simulink model "main"  (R2022a)
settings: Solver=FixedStepDiscrete  StartTime=0.0  StopTime=Inf  FixedStep=(50e-6)-(sim_en*4.995e-5)  RelTol=1e-3  EnableMultiTasking=on
model workspace (MAT data in the model file):
  Param : Simulink.Parameter (value not decoded)
  ac_ok : Simulink.Signal (value not decoded)
  ac_ok_120 : Simulink.Signal (value not decoded)
  bulk_voltage : Simulink.Signal (value not decoded)
  burstduty_integ_max : Simulink.Signal (value not decoded)
  burstduty_integ_min : Simulink.Signal (value not decoded)
  burstduty_ki : Simulink.Signal (value not decoded)
  burstduty_kp : Simulink.Signal (value not decoded)
  calib_ok : Simulink.Signal (value not decoded)
  can_addr1 : Simulink.Signal (value not decoded)
  can_addr2 : Simulink.Signal (value not decoded)
  can_addr3 : Simulink.Signal (value not decoded)
  can_addr4 : Simulink.Signal (value not decoded)
  can_data_rx : Simulink.Signal (value not decoded)
  can_data_tx : Simulink.Signal (value not decoded)
  can_timeout_120 : Simulink.Signal (value not decoded)
  chksum_scircv : Simulink.Signal (value not decoded)
  clllc_en_120 : Simulink.Signal (value not decoded)
  clllc_fault_120 : Simulink.Signal (value not decoded)
  clllc_ok_120 : Simulink.Signal (value not decoded)
  cmpss1h : Simulink.Signal (value not decoded)
  cmpss1l : Simulink.Signal (value not decoded)
  cmpss2h : Simulink.Signal (value not decoded)
  cmpss2l : Simulink.Signal (value not decoded)
  cmpss3h : Simulink.Signal (value not decoded)
  cmpss3l : Simulink.Signal (value not decoded)
  cmpss4h : Simulink.Signal (value not decoded)
  cmpss4l : Simulink.Signal (value not decoded)
  cmpss5h : Simulink.Signal (value not decoded)
  cmpss5l : Simulink.Signal (value not decoded)
  cmpss6h : Simulink.Signal (value not decoded)
  cmpss6l : Simulink.Signal (value not decoded)
  cmpss7h : Simulink.Signal (value not decoded)
  cmpss7l : Simulink.Signal (value not decoded)
  cmpss8h : Simulink.Signal (value not decoded)
  cmpss8l : Simulink.Signal (value not decoded)
  cnt_idle : Simulink.Signal (value not decoded)
  cnt_orps : Simulink.Signal (value not decoded)
  cnt_scircv : Simulink.Signal (value not decoded)
  cnt_scixmt : Simulink.Signal (value not decoded)
  cnt_scixmt_func : Simulink.Signal (value not decoded)
  cnt_temp_mux : Simulink.Signal (value not decoded)
  cnt_vdroop : Simulink.Signal (value not decoded)
  config_ok : Simulink.Signal (value not decoded)
  control_en : Simulink.Signal (value not decoded)
  cp_ready_120 : Simulink.Signal (value not decoded)
  d2d_en : Simulink.Signal (value not decoded)
  dchg_off : Simulink.Signal (value not decoded)
  debug_dacb : Simulink.Signal (value not decoded)
  debug_dacc : Simulink.Signal (value not decoded)
  debug_msg1 : Simulink.Signal (value not decoded)
  debug_msg2 : Simulink.Signal (value not decoded)
  debug_msg3 : Simulink.Signal (value not decoded)
  debug_msg4 : Simulink.Signal (value not decoded)
  debug_msg5 : Simulink.Signal (value not decoded)
  debug_msg6 : Simulink.Signal (value not decoded)
  dir_v2g : Simulink.Signal (value not decoded)
  eoss_llc1 : Simulink.Signal (value not decoded)
  eoss_llc2 : Simulink.Signal (value not decoded)
  eoss_orps : Simulink.Signal (value not decoded)
  fault_ocp : Simulink.Signal (value not decoded)
  fault_otp : Simulink.Signal (value not decoded)
  fault_ovp : Simulink.Signal (value not decoded)
  fut_en : Simulink.Signal (value not decoded)
  fwd_en_120 : Simulink.Signal (value not decoded)
  gain_llc1_sec_idc : Simulink.Signal (value not decoded)
  gain_llc1_temp_sr : Simulink.Signal (value not decoded)
  gain_llc2_sec_idc : Simulink.Signal (value not decoded)
  gain_vbat : Simulink.Signal (value not decoded)
  gain_vbulk : Simulink.Signal (value not decoded)
  gain_vout : Simulink.Signal (value not decoded)
  input_current_phasea : Simulink.Signal (value not decoded)
  input_current_phaseb : Simulink.Signal (value not decoded)
  input_current_phasec : Simulink.Signal (value not decoded)
  input_freq : Simulink.Signal (value not decoded)
  input_power : Simulink.Signal (value not decoded)
  input_voltage_phasea : Simulink.Signal (value not decoded)
  input_voltage_phaseb : Simulink.Signal (value not decoded)
  input_voltage_phasec : Simulink.Signal (value not decoded)
  ishare_arbiter : Simulink.Signal (value not decoded)
  ishare_thresh : Simulink.Signal (value not decoded)
  led_g : Simulink.Signal (value not decoded)
  led_r : Simulink.Signal (value not decoded)
  led_y : Simulink.Signal (value not decoded)
  llc1_burst_integ : Simulink.Signal (value not decoded)
  llc1_burstduty_buffer : Simulink.Signal (value not decoded)
  llc1_pfm_error : Simulink.Signal (value not decoded)
  llc1_pfm_integ : Simulink.Signal (value not decoded)
  llc1_pfm_prop : Simulink.Signal (value not decoded)
  llc1_pri_idc : Simulink.Signal (value not decoded)
  llc1_ps_buffer : Simulink.Signal (value not decoded)
  llc1_pspwm_error : Simulink.Signal (value not decoded)
  llc1_pspwm_integ : Simulink.Signal (value not decoded)
  llc1_pspwm_prop : Simulink.Signal (value not decoded)
  llc1_sec_idc : Simulink.Signal (value not decoded)
  llc1_temp_sr : Simulink.Signal (value not decoded)
  llc1_ts_tbctr_buffer : Simulink.Signal (value not decoded)
  llc2_burst_integ : Simulink.Signal (value not decoded)
  llc2_burstduty_buffer : Simulink.Signal (value not decoded)
  llc2_en : Simulink.Signal (value not decoded)
  llc2_en_buffer : Simulink.Signal (value not decoded)
  llc2_pfm_error : Simulink.Signal (value not decoded)
  llc2_pfm_integ : Simulink.Signal (value not decoded)
  llc2_pfm_prop : Simulink.Signal (value not decoded)
  llc2_pri_idc : Simulink.Signal (value not decoded)
  llc2_ps_buffer : Simulink.Signal (value not decoded)
  llc2_pspwm_error : Simulink.Signal (value not decoded)
  llc2_pspwm_integ : Simulink.Signal (value not decoded)
  llc2_pspwm_prop : Simulink.Signal (value not decoded)
  llc2_sec_idc : Simulink.Signal (value not decoded)
  llc2_temp_sr : Simulink.Signal (value not decoded)
  llc2_ts_tbctr_buffer : Simulink.Signal (value not decoded)
  loop_adcint : Simulink.Signal (value not decoded)
  loop_control : Simulink.Signal (value not decoded)
  loop_idle : Simulink.Signal (value not decoded)
  mid_bulk_voltage : Simulink.Signal (value not decoded)
  mode_120 : Simulink.Signal (value not decoded)
  mode_cc_cv : Simulink.Signal (value not decoded)
  myParam : mpt.Parameter (value not decoded)
  obc_ok_120 : Simulink.Signal (value not decoded)
  offset_llc1_sec_idc : Simulink.Signal (value not decoded)
  offset_llc1_temp_sr : Simulink.Signal (value not decoded)
  offset_llc2_sec_idc : Simulink.Signal (value not decoded)
  offset_vbat : Simulink.Signal (value not decoded)
  offset_vbulk : Simulink.Signal (value not decoded)
  offset_vout : Simulink.Signal (value not decoded)
  openloop_en : Simulink.Signal (value not decoded)
  openloop_fault_en : Simulink.Signal (value not decoded)
  ot_fault_120 : Simulink.Signal (value not decoded)
  pfc_en : Simulink.Signal (value not decoded)
  pfc_en_120 : Simulink.Signal (value not decoded)
  pfc_fw_revision : Simulink.Signal (value not decoded)
  pfc_fw_revision_bootloader : Simulink.Signal (value not decoded)
  pfc_fw_revision_debug : Simulink.Signal (value not decoded)
  pfc_ok : Simulink.Signal (value not decoded)
  pfc_ok_120 : Simulink.Signal (value not decoded)
  pfm_a0 : Simulink.Signal (value not decoded)
  pfm_a1 : Simulink.Signal (value not decoded)
  pfm_integ_max : Simulink.Signal (value not decoded)
  pfm_integ_min : Simulink.Signal (value not decoded)
  pfm_ki : Simulink.Signal (value not decoded)
  pfm_kp : Simulink.Signal (value not decoded)
  pri_fut_en : Simulink.Signal (value not decoded)
  pri_fut_en_buffer : Simulink.Signal (value not decoded)
  pri_halfbridge_en : Simulink.Signal (value not decoded)
  pri_halfbridge_en_buffer : Simulink.Signal (value not decoded)
  pspwm_integ_max : Simulink.Signal (value not decoded)
  pspwm_integ_min : Simulink.Signal (value not decoded)
  pspwm_ki : Simulink.Signal (value not decoded)
  pspwm_kp : Simulink.Signal (value not decoded)
  ref_idclink_max : Simulink.Signal (value not decoded)
  ref_iout : Simulink.Signal (value not decoded)
  ref_iout_calib : Simulink.Signal (value not decoded)
  ref_iout_llc1 : Simulink.Signal (value not decoded)
  ref_iout_llc1_calib : Simulink.Signal (value not decoded)
  ref_iout_llc2 : Simulink.Signal (value not decoded)
  ref_iout_llc2_calib : Simulink.Signal (value not decoded)
  ref_pout : Simulink.Signal (value not decoded)
  ref_ss_llc1 : Simulink.Signal (value not decoded)
  ref_ss_llc2 : Simulink.Signal (value not decoded)
  ref_ss_orps : Simulink.Signal (value not decoded)
  ref_vbat : Simulink.Signal (value not decoded)
  ref_vbat_calib : Simulink.Signal (value not decoded)
  ref_vbulk : Simulink.Signal (value not decoded)
  ref_vbulk_calib : Simulink.Signal (value not decoded)
  ref_vbulk_llc1_calib : Simulink.Signal (value not decoded)
  ref_vbulk_llc2_calib : Simulink.Signal (value not decoded)
  ref_vout : Simulink.Signal (value not decoded)
  ref_vout_calib : Simulink.Signal (value not decoded)
  relay_en : Simulink.Signal (value not decoded)
  reset_flag : Simulink.Signal (value not decoded)
  rev_en_120 : Simulink.Signal (value not decoded)
  runtime_control : Simulink.Signal (value not decoded)
  runtime_idle : Simulink.Signal (value not decoded)
  scircv_buffer : Simulink.Signal (value not decoded)
  scircv_buffer_tmp : Simulink.Signal (value not decoded)
  scircv_buffer_tmp_idx0 : Simulink.Signal (value not decoded)
  scircv_chksum : Simulink.Signal (value not decoded)
  scircv_chksum_ok : Simulink.Signal (value not decoded)
  scircv_parse_ok : Simulink.Signal (value not decoded)
  scixmt_buffer : Simulink.Signal (value not decoded)
  scixmt_chksum : Simulink.Signal (value not decoded)
  scixmt_func : Simulink.Signal (value not decoded)
  scixmt_word0_lsb : Simulink.Signal (value not decoded)
  scixmt_word0_msb : Simulink.Signal (value not decoded)
  scixmt_word1_lsb : Simulink.Signal (value not decoded)
  scixmt_word1_msb : Simulink.Signal (value not decoded)
  scixmt_word2_lsb : Simulink.Signal (value not decoded)
  scixmt_word2_msb : Simulink.Signal (value not decoded)
  scixmt_wr : Simulink.Signal (value not decoded)
  ss_step : Simulink.Signal (value not decoded)
  state_calib : Simulink.Signal (value not decoded)
  state_control : Simulink.Signal (value not decoded)
  state_hkeep : Simulink.Signal (value not decoded)
  status_cmpss : Simulink.Signal (value not decoded)
  status_control : Simulink.Signal (value not decoded)
  status_digin : Simulink.Signal (value not decoded)
  status_digout : Simulink.Signal (value not decoded)
  status_fault : Simulink.Signal (value not decoded)
  status_input : Simulink.Signal (value not decoded)
  status_pfc : Simulink.Signal (value not decoded)
  temp_inlet : Simulink.Signal (value not decoded)
  temp_llc1_fet_hs : Simulink.Signal (value not decoded)
  temp_llc2_fet_hs : Simulink.Signal (value not decoded)
  temp_mux : Simulink.Signal (value not decoded)
  temp_mux_s0 : Simulink.Signal (value not decoded)
  temp_mux_s1 : Simulink.Signal (value not decoded)
  temp_mux_s2 : Simulink.Signal (value not decoded)
  temp_outlet : Simulink.Signal (value not decoded)
  temp_pfc_fet_hsa : Simulink.Signal (value not decoded)
  temp_pfc_fet_hsb : Simulink.Signal (value not decoded)
  temp_pfc_fet_hsc : Simulink.Signal (value not decoded)
  temp_pfc_fet_lsa : Simulink.Signal (value not decoded)
  temp_pfc_fet_lsb : Simulink.Signal (value not decoded)
  temp_pfc_fet_lsc : Simulink.Signal (value not decoded)
  test_mode : Simulink.Signal (value not decoded)
  tfcv_cc : Simulink.Signal (value not decoded)
  tfcv_cc_llc2 : Simulink.Signal (value not decoded)
  tfcv_cv : Simulink.Signal (value not decoded)
  tfcv_sr_en : Simulink.Signal (value not decoded)
  tfv_assert_llc1_pri_idc : Simulink.Signal (value not decoded)
  tfv_assert_llc1_sec_idc : Simulink.Signal (value not decoded)
  tfv_assert_llc1_temp_sr : Simulink.Signal (value not decoded)
  tfv_assert_llc2_pri_idc : Simulink.Signal (value not decoded)
  tfv_assert_llc2_sec_idc : Simulink.Signal (value not decoded)
  tfv_assert_llc2_temp_sr : Simulink.Signal (value not decoded)
  tfv_assert_temp_outlet : Simulink.Signal (value not decoded)
  tfv_assert_vaux_uv : Simulink.Signal (value not decoded)
  tfv_assert_vbat : Simulink.Signal (value not decoded)
  tfv_assert_vbulk : Simulink.Signal (value not decoded)
  tfv_assert_vout : Simulink.Signal (value not decoded)
  tfv_cnt_tz : Simulink.Signal (value not decoded)
  tfv_deassert_llc1_pri_idc : Simulink.Signal (value not decoded)
  tfv_deassert_llc1_sec_idc : Simulink.Signal (value not decoded)
  tfv_deassert_llc1_temp_sr : Simulink.Signal (value not decoded)
  tfv_deassert_llc2_pri_idc : Simulink.Signal (value not decoded)
  tfv_deassert_llc2_sec_idc : Simulink.Signal (value not decoded)
  tfv_deassert_llc2_temp_sr : Simulink.Signal (value not decoded)
  tfv_deassert_temp_outlet : Simulink.Signal (value not decoded)
  tfv_deassert_vaux_uv : Simulink.Signal (value not decoded)
  tfv_deassert_vbat : Simulink.Signal (value not decoded)
  tfv_deassert_vbulk : Simulink.Signal (value not decoded)
  tfv_deassert_vout : Simulink.Signal (value not decoded)
  tfv_llc1_pri_idc : Simulink.Signal (value not decoded)
  tfv_llc1_sec_idc : Simulink.Signal (value not decoded)
  tfv_llc1_temp_sr : Simulink.Signal (value not decoded)
  tfv_llc2_pri_idc : Simulink.Signal (value not decoded)
  tfv_llc2_sec_idc : Simulink.Signal (value not decoded)
  tfv_llc2_temp_sr : Simulink.Signal (value not decoded)
  tfv_temp_outlet : Simulink.Signal (value not decoded)
  tfv_vaux_uv : Simulink.Signal (value not decoded)
  tfv_vbat : Simulink.Signal (value not decoded)
  tfv_vbulk : Simulink.Signal (value not decoded)
  tfv_vout : Simulink.Signal (value not decoded)
  timer_1ms : Simulink.Signal (value not decoded)
  tz : Simulink.Signal (value not decoded)
  valve_en : Simulink.Signal (value not decoded)
  vaux : Simulink.Signal (value not decoded)
  vbat : Simulink.Signal (value not decoded)
  vbulk : Simulink.Signal (value not decoded)
  vout : Simulink.Signal (value not decoded)
undefined symbols (not defined in the file or in its folder): CAN_O_INT, CANA_BASE, Down, GPTRIP1SEL, GPTRIP2SEL, TZ1, TZ2, Up
libraries: hdlsllib x159, simulink x94, c2802xlib x32, c2837xDlib x19, c2807xlib x16, c280xlib x13, canmsglib x8, idelinklib_common x2, c2000lib x1, c281xlib x1
(part 2 of 20)

== system main/Control_State_Machine/control/disClb ==
  note: //disable CLB
      | CLB_disableCLB(CLB1_BASE);
      | CLB_disableCLB(CLB2_BASE);
      |
      | //disable xbar clb mux
      | //G2V
      | XBAR_disableCLBMux(XBAR_AUXSIG0, XBAR_MUX08);
      | XBAR_disableCLBMux(XBAR_AUXSIG1, XBAR_MUX09);
      | XBAR_disableCLBMux(XBAR_AUXSIG2, XBAR_MUX10);
      | XBAR_disableCLBMux(XBAR_AUXSIG3, XBAR_MUX11);
      |
      | //V2G
      | XBAR_disableCLBMux(XBAR_AUXSIG0, XBAR_MUX00);
      | XBAR_disableCLBMux(XBAR_AUXSIG1, XBAR_MUX01);
      | XBAR_disableCLBMux(XBAR_AUXSIG2, XBAR_MUX02);
      | XBAR_disableCLBMux(XBAR_AUXSIG3, XBAR_MUX03);
      |
      |
      | //disable xbar epwm mux
      | //G2V
      | XBAR_disableEPWMMux(XBAR_TRIP9, XBAR_MUX05);
      | XBAR_disableEPWMMux(XBAR_TRIP10, XBAR_MUX01);
      |
      | //V2G
      | XBAR_disableEPWMMux(XBAR_TRIP4, XBAR_MUX05);
      | XBAR_disableEPWMMux(XBAR_TRIP5, XBAR_MUX01);
  f : TriggerPort  TriggerType=function-call  VariantControl=(inherit)
      settings: CopyFcn=Stateflow.SLINSF.SimulinkMan.removeBlockPreDeleteFcn  PreDeleteFcn=Stateflow.SLINSF.SimulinkMan.unsafePredeleteFcn
  System Outputs1 : Subsystem  mask(System Outputs){ShowInLibBrowser=0}
      mask prompts: ShowInLibBrowser "Simulink:masks:CustCodeMaskParam1_MP"
      settings: CopyFcn=cccopyfcn(gcb)  OpenFcn=ccopenfcn('System Outputs Function')
      mask Help: eval('feval(''rtwprivate'',''rtwhelpview'',''rtw_sys_outputs_block'')');
      mask Display: disp('System\nOutputs');

== system main/Control_State_Machine/control/disPwm ==
  note: Note:
      | at the start, all 16 pwms are configured AQ, force LOW
  note: Sequence:
      | 1.) AQCSFRC all 16 pwm
      | 2.) Disable all epwm trip
  note: Reset:
      | integ_
      | integ_
      | ts_
      | ts_
  f : TriggerPort  TriggerType=function-call  VariantControl=(inherit)
      settings: CopyFcn=Stateflow.SLINSF.SimulinkMan.removeBlockPreDeleteFcn  PreDeleteFcn=Stateflow.SLINSF.SimulinkMan.unsafePredeleteFcn
  disPwm : Subsystem  Variant=on

== system main/Control_State_Machine/control/disableSR ==
  note: //EPwm1Regs.AQCSFRC.bit.CSFA = 0b0; //force disable
      | //EPwm1Regs.AQCSFRC.bit.CSFB = 0b0; //force disable
      | //EPwm2Regs.AQCSFRC.bit.CSFA = 0b0; //force disable
      | //EPwm2Regs.AQCSFRC.bit.CSFB = 0b0; //force disable
      | EPwm7Regs.AQCSFRC.bit.CSFA = 0b1; //force low
      | EPwm7Regs.AQCSFRC.bit.CSFB = 0b1; //force low
      | EPwm8Regs.AQCSFRC.bit.CSFA = 0b1; //force low
      | EPwm8Regs.AQCSFRC.bit.CSFB = 0b1; //force low
  f : TriggerPort  TriggerType=function-call  VariantControl=(inherit)
      settings: CopyFcn=Stateflow.SLINSF.SimulinkMan.removeBlockPreDeleteFcn  PreDeleteFcn=Stateflow.SLINSF.SimulinkMan.unsafePredeleteFcn
  System Outputs1 : Subsystem  mask(System Outputs){ShowInLibBrowser=0}
      mask prompts: ShowInLibBrowser "Simulink:masks:CustCodeMaskParam1_MP"
      settings: CopyFcn=cccopyfcn(gcb)  OpenFcn=ccopenfcn('System Outputs Function')
      mask Help: eval('feval(''rtwprivate'',''rtwhelpview'',''rtw_sys_outputs_block'')');
      mask DialogControl ShowInLibBrowser Prompt: Mask Parameter 1:
      mask Display: disp('System\nOutputs');

== system main/Control_State_Machine/control/enableSR ==
  note: //EPwm1Regs.AQCSFRC.bit.CSFA = 0b0; //force disabled
      | //EPwm1Regs.AQCSFRC.bit.CSFB = 0b0; //force disabled
      | //EPwm2Regs.AQCSFRC.bit.CSFA = 0b0; //force disabled
      | //EPwm2Regs.AQCSFRC.bit.CSFB = 0b0; //force disabled
      |
      | //Enable sync  rec
      | EPwm7Regs.AQCSFRC.bit.CSFA = 0b0; //force disabled
      | EPwm7Regs.AQCSFRC.bit.CSFB = 0b0; //force disabled
      | EPwm8Regs.AQCSFRC.bit.CSFA = 0b0; //force disabled
      | EPwm8Regs.AQCSFRC.bit.CSFB = 0b0; //force disabled
      |
      | //Disable sync rec
      | //EPwm7Regs.AQCSFRC.bit.CSFA = 0b1; //force low
      | //EPwm7Regs.AQCSFRC.bit.CSFB = 0b1; //force low
      | //EPwm8Regs.AQCSFRC.bit.CSFA = 0b1; //force low
      | //EPwm8Regs.AQCSFRC.bit.CSFB = 0b1; //force low
  f : TriggerPort  TriggerType=function-call  VariantControl=(inherit)
      settings: CopyFcn=Stateflow.SLINSF.SimulinkMan.removeBlockPreDeleteFcn  PreDeleteFcn=Stateflow.SLINSF.SimulinkMan.unsafePredeleteFcn
  System Outputs : Subsystem  mask(System Outputs){ShowInLibBrowser=0}
      mask prompts: ShowInLibBrowser "Simulink:masks:CustCodeMaskParam1_MP"
      settings: CopyFcn=cccopyfcn(gcb)  OpenFcn=ccopenfcn('System Outputs Function')
      mask Help: eval('feval(''rtwprivate'',''rtwhelpview'',''rtw_sys_outputs_block'')');
      mask DialogControl ShowInLibBrowser Prompt: Mask Parameter 1:
      mask Display: disp('System\nOutputs');
  enPwm : Subsystem  Commented=on  Variant=on

== system main/Control_State_Machine/control/initG2vCcBurst ==
  f : TriggerPort  TriggerType=function-call  VariantControl=(inherit)
      settings: CopyFcn=Stateflow.SLINSF.SimulinkMan.removeBlockPreDeleteFcn  PreDeleteFcn=Stateflow.SLINSF.SimulinkMan.unsafePredeleteFcn
  initG2vCcBurst : Subsystem  Variant=on

== system main/Control_State_Machine/control/initG2vCcPfm ==
  f : TriggerPort  TriggerType=function-call  VariantControl=(inherit)
      settings: CopyFcn=Stateflow.SLINSF.SimulinkMan.removeBlockPreDeleteFcn  PreDeleteFcn=Stateflow.SLINSF.SimulinkMan.unsafePredeleteFcn
  initG2vCcPfm : Subsystem  Variant=on

== system main/Control_State_Machine/control/initG2vCcPspwm ==
  f : TriggerPort  TriggerType=function-call  VariantControl=(inherit)
      settings: CopyFcn=Stateflow.SLINSF.SimulinkMan.removeBlockPreDeleteFcn  PreDeleteFcn=Stateflow.SLINSF.SimulinkMan.unsafePredeleteFcn
  initG2vCcPfm : Subsystem  Variant=on

== system main/Control_State_Machine/control/initG2vCvBurst ==
  f : TriggerPort  TriggerType=function-call  VariantControl=(inherit)
      settings: CopyFcn=Stateflow.SLINSF.SimulinkMan.removeBlockPreDeleteFcn  PreDeleteFcn=Stateflow.SLINSF.SimulinkMan.unsafePredeleteFcn
  initG2vCvBurst : Subsystem  Variant=on

== system main/Control_State_Machine/control/initG2vCvPfm ==
  f : TriggerPort  TriggerType=function-call  VariantControl=(inherit)
      settings: CopyFcn=Stateflow.SLINSF.SimulinkMan.removeBlockPreDeleteFcn  PreDeleteFcn=Stateflow.SLINSF.SimulinkMan.unsafePredeleteFcn
  initG2vCvPfm : Subsystem  Variant=on

== system main/Control_State_Machine/control/initG2vCvPspwm ==
  f : TriggerPort  TriggerType=function-call  VariantControl=(inherit)
      settings: CopyFcn=Stateflow.SLINSF.SimulinkMan.removeBlockPreDeleteFcn  PreDeleteFcn=Stateflow.SLINSF.SimulinkMan.unsafePredeleteFcn
  initG2vCvPfm : Subsystem  Variant=on

== system main/Control_State_Machine/control/initV2gCvBurst ==
  f : TriggerPort  TriggerType=function-call  VariantControl=(inherit)
      settings: CopyFcn=Stateflow.SLINSF.SimulinkMan.removeBlockPreDeleteFcn  PreDeleteFcn=Stateflow.SLINSF.SimulinkMan.unsafePredeleteFcn
  initV2gCvBurst : Subsystem  Variant=on

== system main/Control_State_Machine/control/initV2gCvPfm ==
  f : TriggerPort  TriggerType=function-call  VariantControl=(inherit)
      settings: CopyFcn=Stateflow.SLINSF.SimulinkMan.removeBlockPreDeleteFcn  PreDeleteFcn=Stateflow.SLINSF.SimulinkMan.unsafePredeleteFcn
  initV2gCvPfm : Subsystem  Variant=on

== system main/Control_State_Machine/control/initV2gCvPspwm ==
  f : TriggerPort  TriggerType=function-call  VariantControl=(inherit)
      settings: CopyFcn=Stateflow.SLINSF.SimulinkMan.removeBlockPreDeleteFcn  PreDeleteFcn=Stateflow.SLINSF.SimulinkMan.unsafePredeleteFcn
  initV2gCvPspwm : Subsystem  Variant=on

== system main/Control_State_Machine/control/openloopControlParam ==
  f : TriggerPort  TriggerType=function-call  VariantControl=(inherit)
      settings: CopyFcn=Stateflow.SLINSF.SimulinkMan.removeBlockPreDeleteFcn  PreDeleteFcn=Stateflow.SLINSF.SimulinkMan.unsafePredeleteFcn
  Data Store Read1 : DataStoreRead  DataStoreName=f32PhaseShift1  IndexOptions=Index vector (dialog)  Indices=1  OutputSizes=1
  Data Store Read2 : DataStoreRead  DataStoreName=f32FreqPeriod1  IndexOptions=Index vector (dialog)  Indices=1  OutputSizes=1
  Data Store Read3 : DataStoreRead  DataStoreName=f32BurstDuty1  IndexOptions=Index vector (dialog)  Indices=1  OutputSizes=1
  FreqPeriod1 : Outport
  PhaseShift1 : Outport  Port=2
  BurstDuty1 : Outport  Port=3
  wires:
  Data Store Read2/1 -> FreqPeriod1/1
  Data Store Read1/1 -> PhaseShift1/1
  Data Store Read3/1 -> BurstDuty1/1

== system main/Control_State_Machine/control/pfmLlc1 ==
  note: Compensation:
  ref : Inport
  input : Inport  Port=2
  pfm_integ_in : Inport  Port=3
  f : TriggerPort  TriggerType=function-call  VariantControl=(inherit)
      settings: CopyFcn=Stateflow.SLINSF.SimulinkMan.removeBlockPreDeleteFcn  PreDeleteFcn=Stateflow.SLINSF.SimulinkMan.unsafePredeleteFcn
  Data Store Read : DataStoreRead  DataStoreName=pfm_kp  IndexOptions=Index vector (dialog)  Indices=1  OutputSizes=1
  Data Store Read2 : DataStoreRead  DataStoreName=pfm_ki  IndexOptions=Index vector (dialog)  Indices=1  OutputSizes=1
  Data Store Read3 : DataStoreRead  DataStoreName=pfm_integ_max  IndexOptions=Index vector (dialog)  Indices=1  OutputSizes=1
  Data Store Read4 : DataStoreRead  DataStoreName=pfm_integ_min  IndexOptions=Index vector (dialog)  Indices=1  OutputSizes=1
  Data Type Conversion : DataTypeConversion  OutDataTypeStr=single  SaturateOnIntegerOverflow=off  RndMeth=Floor
  Delay1 : Delay  DelayLength=1  InitialCondition=0
  Gain3 : Gain  Gain=-1
  Product : Product
  Product1 : Product
  Saturation Dynamic3 : simulink/Discontinuities/Saturation Dynamic  OutMin=[]  OutMax=[]  OutDataTypeStr=double  OutputDataTypeScalingMode=double  OutDataType=fixdt(1, 16)  OutScaling=2^-10  DoSatur=off
  Sum5 : Sum  Inputs=++-
  Sum6 : Sum  Inputs=|+-
  llc1_ts_tbctr : Outport
  wires:
  ref/1 -> Sum6/1
  Data Store Read2/1 -> [a1]
  Data Store Read3/1 -> [integ_max]
  Data Store Read4/1 -> [integ_min]
  Data Type Conversion/1 -> [error]
  Data Store Read/1 -> [a0]
  Sum6/1 -> Data Type Conversion/1
  input/1 -> Sum6/2
  Product/1 -> Sum5/2
  [error] -> Delay1/1, Product1/1  "Error"
  [integ_max] -> Saturation Dynamic3/1
  Sum5/1 -> Saturation Dynamic3/2
  Saturation Dynamic3/1 -> llc1_ts_tbctr/1
  Delay1/1 -> Product/1
  Gain3/1 -> Sum5/3
  [integ_min] -> Saturation Dynamic3/3
  Product1/1 -> Sum5/1
  [a0] -> Product1/2
  [a1] -> Product/2
  pfm_integ_in/1 -> Gain3/1

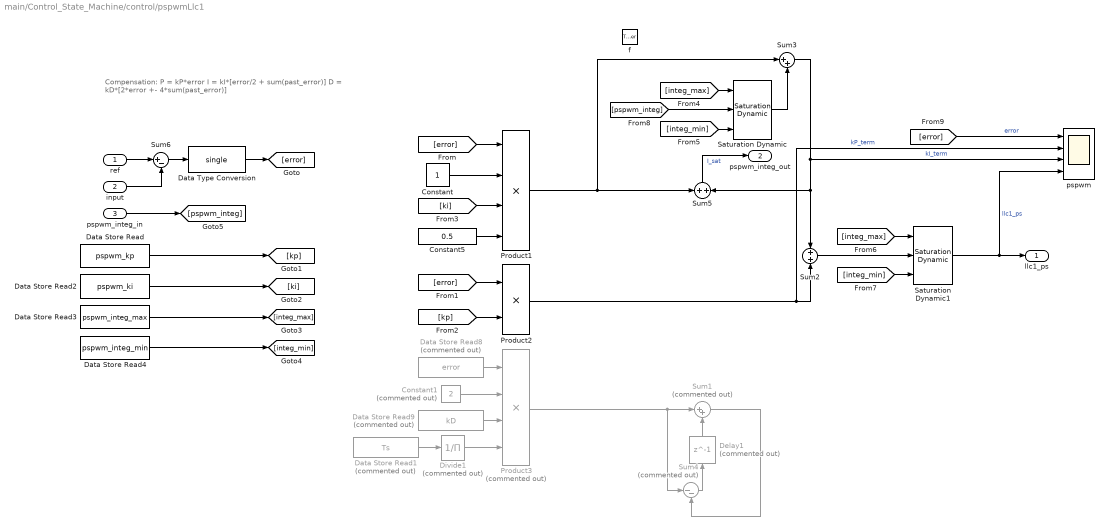
== system main/Control_State_Machine/control/pspwmLlc1 ==
  note: Compensation:
      | P = kP*error
      | I = kI*[error/2 + sum(past_error)]
      | D = kD*[2*error +- 4*sum(past_error)]
  ref : Inport
  input : Inport  Port=2
  pspwm_integ_in : Inport  Port=3
  f : TriggerPort  TriggerType=function-call  VariantControl=(inherit)
      settings: CopyFcn=Stateflow.SLINSF.SimulinkMan.removeBlockPreDeleteFcn  PreDeleteFcn=Stateflow.SLINSF.SimulinkMan.unsafePredeleteFcn
  Constant : Constant  OutDataTypeStr=single
  Constant1 : Constant  Commented=on  Value=2  OutDataTypeStr=single
  Constant5 : Constant  Value=0.5  OutDataTypeStr=single
  Data Store Read : DataStoreRead  DataStoreName=pspwm_kp  IndexOptions=Index vector (dialog)  Indices=1  OutputSizes=1
  Data Store Read1 : DataStoreRead  Commented=on  DataStoreName=Ts  IndexOptions=Index vector (dialog)  Indices=1  OutputSizes=1
  Data Store Read2 : DataStoreRead  DataStoreName=pspwm_ki  IndexOptions=Index vector (dialog)  Indices=1  OutputSizes=1
  Data Store Read3 : DataStoreRead  DataStoreName=pspwm_integ_max  IndexOptions=Index vector (dialog)  Indices=1  OutputSizes=1
  Data Store Read4 : DataStoreRead  DataStoreName=pspwm_integ_min  IndexOptions=Index vector (dialog)  Indices=1  OutputSizes=1
  Data Store Read8 : DataStoreRead  Commented=on  DataStoreName=error  IndexOptions=Index vector (dialog)  Indices=1  OutputSizes=1
  Data Store Read9 : DataStoreRead  Commented=on  DataStoreName=kD  IndexOptions=Index vector (dialog)  Indices=1  OutputSizes=1
  Data Type Conversion : DataTypeConversion  OutDataTypeStr=single  SaturateOnIntegerOverflow=off  RndMeth=Floor
  Delay1 : Delay  Commented=on  DelayLength=1  InitialCondition=310  StateName=deriv_delay
  Divide1 : Product  Commented=on  Inputs=/
  Product1 : Product  Inputs=4
  Product2 : Product
  Product3 : Product  Commented=on  Inputs=4
  Saturation Dynamic : simulink/Discontinuities/Saturation Dynamic  OutMin=[]  OutMax=[]  OutDataTypeStr=single  OutputDataTypeScalingMode=single  OutDataType=fixdt(1, 16)  OutScaling=2^-10  DoSatur=off
  Saturation Dynamic1 : simulink/Discontinuities/Saturation Dynamic  OutMin=[]  OutMax=[]  OutDataTypeStr=single  OutputDataTypeScalingMode=single  OutDataType=fixdt(1, 16)  OutScaling=2^-10  DoSatur=off
  Sum1 : Sum  Commented=on  Inputs=|++
  Sum2 : Sum  Inputs=2
  Sum3 : Sum  Inputs=|++
  Sum4 : Sum  Commented=on  Inputs=|--
  Sum5 : Sum  Inputs=2
  Sum6 : Sum  Inputs=|+-
  pspwm : Scope  NumInputPorts=4
  llc1_ps : Outport
  pspwm_integ_out : Outport  Port=2
  wires:
  Constant/1 -> Product1/2
  Data Store Read/1 -> [kp]
  Data Store Read2/1 -> [ki]
  Sum6/1 -> Data Type Conversion/1
  Data Type Conversion/1 -> [error]
  Data Store Read4/1 -> [integ_min]
  Data Store Read3/1 -> [integ_max]
  input/1 -> Sum6/2
  ref/1 -> Sum6/1
  Data Store Read1/1 -> Divide1/1
  Sum4/1 -> Delay1/1
  [integ_max] -> Saturation Dynamic1/1
  [error] -> Product2/1
  [ki] -> Product1/3
  Saturation Dynamic/1 -> Sum3/2
  Saturation Dynamic1/1 -> pspwm/4, llc1_ps/1  "llc1_ps"
  [integ_min] -> Saturation Dynamic1/3
  Data Store Read9/1 -> Product3/3
  [integ_max] -> Saturation Dynamic/1
  Data Store Read8/1 -> Product3/1
  Sum3/1 -> pspwm/3, Sum2/1, Sum5/2  "kI_term"
  Product2/1 -> pspwm/2, Sum2/2  "kP_term"
  Divide1/1 -> Product3/4
  [integ_min] -> Saturation Dynamic/3
  Constant5/1 -> Product1/4
  Sum2/1 -> Saturation Dynamic1/2
  Product3/1 -> Sum1/1, Sum4/1
  Constant1/1 -> Product3/2
  [error] -> Product1/1
  Sum1/1 -> Sum4/2
  [kp] -> Product2/2
  Product1/1 -> Sum5/1, Sum3/1
  Delay1/1 -> Sum1/2
  [error] -> pspwm/1  "error"
  pspwm_integ_in/1 -> [pspwm_integ]
  [pspwm_integ] -> Saturation Dynamic/2
  Sum5/1 -> pspwm_integ_out/1  "I_sat"

== system main/Control_State_Machine/control/resetControlParam ==
  dir_v2g : Inport
  f : TriggerPort  TriggerType=function-call  VariantControl=(inherit)
      settings: CopyFcn=Stateflow.SLINSF.SimulinkMan.removeBlockPreDeleteFcn  PreDeleteFcn=Stateflow.SLINSF.SimulinkMan.unsafePredeleteFcn
  If : If  IfExpression=(u1==0)
  g2v_prifullbridge : Subsystem  TreatAsAtomicUnit=on
  v2g_prifullbridge : Subsystem  TreatAsAtomicUnit=on
  wires:
  dir_v2g/1 -> If/1
  If/1 -> g2v_prifullbridge/Action
  If/2 -> v2g_prifullbridge/Action

== system main/Control_State_Machine/control/tfcvCc ==
  input : Inport  OutDataTypeStr=uint16  PortDimensions=1
  assert_lim : Inport  Port=2  OutDataTypeStr=uint16  PortDimensions=1
  assert_vld : Inport  Port=3  OutDataTypeStr=uint16  PortDimensions=1
  deassert_lim : Inport  Port=4  OutDataTypeStr=uint16  PortDimensions=1
  deassert_vld : Inport  Port=5  OutDataTypeStr=uint16  PortDimensions=1
  f : TriggerPort  TriggerType=function-call  VariantControl=(inherit)
      settings: CopyFcn=Stateflow.SLINSF.SimulinkMan.removeBlockPreDeleteFcn  PreDeleteFcn=Stateflow.SLINSF.SimulinkMan.unsafePredeleteFcn
  Data Type Conversion : DataTypeConversion  OutDataTypeStr=boolean  SaturateOnIntegerOverflow=off  RndMeth=Floor
  tfcv : MATLABSystem  System=tfcv  SimulateUsing=Code generation
      mask Type: tfcv
      mask Display:
      | disp('tfcv');
      | port_label('input',1,'input');
      | port_label('input',2,'assert_lim');
      | port_label('input',3,'assert_vld');
      | port_label('input',4,'deassert_lim');
      | port_label('input',5,'deassert_vld');
      | port_label('output',1,'status');
  tfv_status : Outport  OutDataTypeStr=boolean
  wires:
  deassert_vld/1 -> tfcv/5
  deassert_lim/1 -> tfcv/4
  assert_vld/1 -> tfcv/3
  assert_lim/1 -> tfcv/2
  input/1 -> tfcv/1
  tfcv/1 -> Data Type Conversion/1
  Data Type Conversion/1 -> tfv_status/1

== system main/Control_State_Machine/control/tfcvCv ==
  input : Inport  OutDataTypeStr=uint16  PortDimensions=1
  assert_lim : Inport  Port=2  OutDataTypeStr=uint16  PortDimensions=1
  assert_vld : Inport  Port=3  OutDataTypeStr=uint16  PortDimensions=1
  deassert_lim : Inport  Port=4  OutDataTypeStr=uint16  PortDimensions=1
  deassert_vld : Inport  Port=5  OutDataTypeStr=uint16  PortDimensions=1
  f : TriggerPort  TriggerType=function-call  VariantControl=(inherit)
      settings: CopyFcn=Stateflow.SLINSF.SimulinkMan.removeBlockPreDeleteFcn  PreDeleteFcn=Stateflow.SLINSF.SimulinkMan.unsafePredeleteFcn
  Data Type Conversion : DataTypeConversion  OutDataTypeStr=boolean  SaturateOnIntegerOverflow=off  RndMeth=Floor
  tfcv : MATLABSystem  System=tfcv  SimulateUsing=Code generation
      mask Type: tfcv
      mask Display:
      | disp('tfcv');
      | port_label('input',1,'input');
      | port_label('input',2,'assert_lim');
      | port_label('input',3,'assert_vld');
      | port_label('input',4,'deassert_lim');
      | port_label('input',5,'deassert_vld');
      | port_label('output',1,'status');
  tfv_status : Outport  OutDataTypeStr=boolean
  wires:
  Data Type Conversion/1 -> tfv_status/1
  tfcv/1 -> Data Type Conversion/1
  deassert_vld/1 -> tfcv/5
  deassert_lim/1 -> tfcv/4
  assert_vld/1 -> tfcv/3
  assert_lim/1 -> tfcv/2
  input/1 -> tfcv/1

== system main/Control_State_Machine/control/tzClear ==
  note: EALLOW;
      | EPwm1Regs.TZCLR.bit.OST = 0b1; //clear trip condition
      | EPwm2Regs.TZCLR.bit.OST = 0b1; //clear trip condition
      |
      | EPwm7Regs.TZCLR.bit.OST = 0b1; //clear trip condition
      | EPwm8Regs.TZCLR.bit.OST = 0b1; //clear trip condition
      |
      | EPwm1Regs.TZOSTCLR.bit.OST3 = 0b1; //clear tz flag
      | EDIS;
  f : TriggerPort  TriggerType=function-call  VariantControl=(inherit)
      settings: CopyFcn=Stateflow.SLINSF.SimulinkMan.removeBlockPreDeleteFcn  PreDeleteFcn=Stateflow.SLINSF.SimulinkMan.unsafePredeleteFcn
  System Outputs : Subsystem  mask(System Outputs){ShowInLibBrowser=0}
      mask prompts: ShowInLibBrowser "Simulink:masks:CustCodeMaskParam1_MP"
      settings: CopyFcn=cccopyfcn(gcb)  OpenFcn=ccopenfcn('System Outputs Function')
      mask Help: eval('feval(''rtwprivate'',''rtwhelpview'',''rtw_sys_outputs_block'')');
      mask Display: disp('System\nOutputs');

== system main/Task_Manager/Tmr_1mS ==
  note: 1) Add Subsystem or Model blocks as valid variant choices.
      | 2) You cannot connect blocks at this level. At simulation, connectivity is automatically
      | determined, based on the active variant and port name matching.
  codegen : Subsystem  VariantControl=sim_en==0
  sim : Subsystem  VariantControl=sim_en==1

== system main/Task_Manager/Tmr_1s ==
  note: 1) Add Subsystem or Model blocks as valid variant choices.
      | 2) You cannot connect blocks at this level. At simulation, connectivity is automatically
      | determined, based on the active variant and port name matching.
  codegen : Subsystem  VariantControl=sim_en==0
  sim : Subsystem  VariantControl=sim_en==1

== system main/Task_Manager/Tmr_20mS ==
  note: 1) Add Subsystem or Model blocks as valid variant choices.
      | 2) You cannot connect blocks at this level. At simulation, connectivity is automatically
      | determined, based on the active variant and port name matching.
  codegen : Subsystem  VariantControl=sim_en==0
  sim : Subsystem  VariantControl=sim_en==1

== system main/Task_Manager/idle ==
  sim_digin : Inport
  function : TriggerPort  TriggerType=function-call  VariantControl=Variant  PortDimensions=1
  Constant7 : Constant  Value=8  OutDataTypeStr=uint16
  Constant8 : Constant  Value=8  OutDataTypeStr=uint16
  Data Store Write7 : DataStoreWrite  DataStoreName=runtime_control  IndexOptions=Index vector (dialog)  Indices=1  OutputSizes=1
  Data Store Write8 : DataStoreWrite  DataStoreName=runtime_idle  IndexOptions=Index vector (dialog)  Indices=1  OutputSizes=1
  Function-Call Generator1 : simulink/Ports & Subsystems/Function-Call Generator  sample_time=-1  numberOfIterations=1  DisallowWideOutput=off
  Function-Call Split1 : FunctionCallSplit  NumOutputPorts=2
  cnt_idle : Subsystem  TreatAsAtomicUnit=on
      settings: RTWSystemCode=Inline
  idle_task : Subsystem  TreatAsAtomicUnit=on
      settings: RTWSystemCode=Inline
  sim_digout : Outport
  wires:
  idle_task/1(sim_digout) -> sim_digout/1
  sim_digin/1 -> idle_task/1(sim_digin)
  Constant8/1 -> Data Store Write8/1
  Constant7/1 -> Data Store Write7/1
  Function-Call Generator1/1 -> Function-Call Split1/1
  Function-Call Split1/1 -> idle_task/Trigger
  Function-Call Split1/2 -> cnt_idle/Trigger

== system main/Task_Manager/init ==
  note: 1) Add Subsystem or Model blocks as valid variant choices.
      | 2) You cannot connect blocks at this level. At simulation, connectivity is automatically
      | determined, based on the active variant and port name matching.
  codegen : Subsystem  VariantControl=sim_en==0
  sim : Subsystem  VariantControl=sim_en==1

== system main/interrupt_adca/burst_control ==
  function : TriggerPort  TriggerType=function-call  VariantControl=Variant
  Constant1 : Constant  Value=[0 7 13 19 25 32 38 44 50 57 63 69 75 82 88 94 100]
  Constant2 : Constant  Value=[0 1 2 3 4 5 6 7 8 9 10 11 12 13 14 15 16]
  Data Store Read2 : DataStoreRead  DataStoreName=llc1_burstduty  IndexOptions=Index vector (dialog)  Indices=1  OutputSizes=1
  Lookup Table Dynamic : simulink/Lookup Tables/Lookup Table Dynamic  LookUpMeth=Use Input Below  OutDataType=fixdt('int8')  OutScaling=[]  OutputDataTypeScalingMode=Specify via dialog  OutDataTypeStr=int8  DoSatur=off
  burst : Stateflow chart  TreatAsAtomicUnit=on
  wires:
  Constant1/1 -> Lookup Table Dynamic/2
  Lookup Table Dynamic/1 -> burst/1(burst_pulses)
  Constant2/1 -> Lookup Table Dynamic/3
  Data Store Read2/1 -> Lookup Table Dynamic/1
